simulink model "q_find_deadzone"  (R2014a)
settings: Solver=ode1  StartTime=0.0  StopTime=inf  FixedStep=0.001  RelTol=1e-3
undefined symbols (not defined in the file or in its folder): HIL
libraries: quarc_library x4
settings Model: SimulationMode=external  ExtModeTrigDuration=30000  Creator=Student  LastModifiedBy=Control_Eng
settings SolverCC: PositivePriorityOrder=on
settings RTWCC: SystemTargetFile=quarc_win64.tlc  TemplateMakefile=quarc_default_tmf  Description=QUARC Win64 Target  ProcessScript=quarc_win64_make_rtw_hook
settings STFCustomTargetCC: CombineOutputUpdateFcns=on  GRTInterface=off
settings GRTTargetCC: ParMdlRefBuildCompliant=off  CompOptLevelCompliant=off  MatFileLogging=off  CPPClassGenCompliant=off  ExtMode=on  ExtModeMexFile=quarc_comm

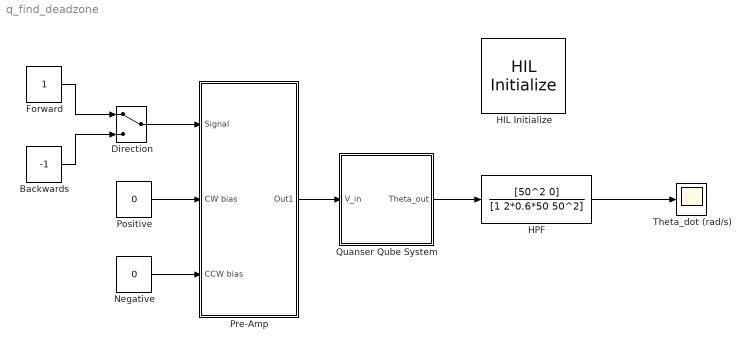
== system q_find_deadzone ==
  Backwards : Constant  Value=-1
  Direction : ManualSwitch
  Forward : Constant
  HIL Initialize : quarc_library/Data Acquisition/Generic/Configuration/HIL Initialize  Priority=-99  object_name=HIL-1  board_type=qube_servo_usb  board_number=0  board_options=d0=pwm;d1=pwm;led=auto;update_rate=normal;decimation=1  exclusive=off  active=off  hardware_clocks=[0]  clock_modes=[]  initial_clock_frequencies=[]  set_clock_params_at_start=off  set_clock_params_at_switch_in=off  set_clock_frequencies_at_start=off  set_clock_frequencies_at_switch_in=off  analog_input_channels=[]  analog_input_maximums=[]  analog_input_minimums=[]  set_analog_input_params_at_start=off  set_analog_input_params_at_switch_in=off  analog_output_channels=[0:1]  analog_output_maximums=10  analog_output_minimums=-10  initial_analog_outputs=[0]  final_analog_outputs=[0]  watchdog_analog_outputs=0  set_analog_output_params_at_start=on  set_analog_output_params_at_switch_in=off  set_analog_outputs_at_start=on  set_analog_outputs_at_switch_in=off  set_analog_outputs_at_terminate=on  set_analog_outputs_at_switch_out=off  set_analog_outputs_on_watchdog=off  digital_input_channels=[]  digital_output_channels=[]  digital_output_configuration=[]  initial_digital_outputs=[]  final_digital_outputs=[]  watchdog_digital_outputs=[]  set_digital_output_params_at_start=off  set_digital_output_params_at_switch_in=off  set_digital_outputs_at_start=off  set_digital_outputs_at_switch_in=off  set_digital_outputs_at_terminate=off  set_digital_outputs_at_switch_out=off  set_digital_outputs_on_watchdog=off  encoder_channels=[0:1]  quadrature=[4]  encoder_filter_frequency=[]  initial_encoder_counts=[0]  set_encoder_params_at_start=on  set_encoder_params_at_switch_in=off  set_encoder_counts_at_start=on  set_encoder_counts_at_switch_in=off  pwm_channels=[]  pwm_modes=[]  pwm_frequency=[]  pwm_configuration=[]  pwm_alignment=[]  pwm_polarity=[]  pwm_leading_deadband=[]  pwm_trailing_deadband=[]  initial_pwm_outputs=[]  final_pwm_outputs=[]  watchdog_pwm_outputs=[]  set_pwm_params_at_start=off  set_pwm_params_at_switch_in=off  set_pwm_outputs_at_start=off  set_pwm_outputs_at_switch_in=off  set_pwm_outputs_at_terminate=off  set_pwm_outputs_at_switch_out=off  set_pwm_outputs_on_watchdog=off  other_output_channels=[]  initial_other_outputs=[]  final_other_outputs=[]  watchdog_other_outputs=[]  set_other_outputs_at_start=off  set_other_outputs_at_switch_in=off  set_other_outputs_at_terminate=off  set_other_outputs_at_switch_out=off  set_other_outputs_on_watchdog=off
  HPF : TransferFcn  Numerator=[50^2 0]  Denominator=[1 2*0.6*50 50^2]
  Negative : Constant  Value=0
  Positive : Constant  Value=0
  Pre-Amp : Subsystem
  Quanser Qube System : Subsystem
  Theta_dot (rad/s) : Scope
      settings: TimeRange=30  YMin=0  YMax=50  SaveName=Output_Data  MaxDataPoints=2500
  wires:
  Quanser Qube System/1(Theta_out) -> HPF/1
  Positive/1 -> Pre-Amp/2(CW bias)
  Negative/1 -> Pre-Amp/3(CCW bias)
  Pre-Amp/1(Out1) -> Quanser Qube System/1(V_in)
  HPF/1 -> Theta_dot (rad/s)/1
  Direction/1 -> Pre-Amp/1(Signal)
  Backwards/1 -> Direction/2
  Forward/1 -> Direction/1

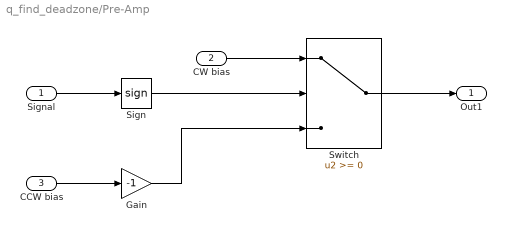
== system q_find_deadzone/Pre-Amp ==
  Signal : Inport
  CW bias : Inport  Port=2
  CCW bias : Inport  Port=3
  Gain : Gain  Gain=-1
  Sign : Signum
  Switch : Switch
  Out1 : Outport
  wires:
  CW bias/1 -> Switch/1
  Signal/1 -> Sign/1
  CCW bias/1 -> Gain/1
  Switch/1 -> Out1/1
  Sign/1 -> Switch/2
  Gain/1 -> Switch/3

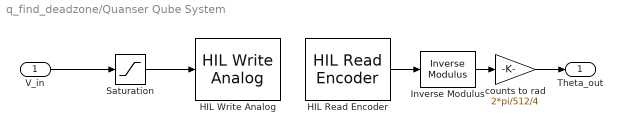
== system q_find_deadzone/Quanser Qube System ==
  V_in : Inport
  HIL Read Encoder : quarc_library/Data Acquisition/Generic/Immediate I//O/HIL Read Encoder  object_name=HIL-1  channels=0  sample_time=qc_get_step_size  active=on  vector_output=off  data_type_mode=Inherit via back propagation  data_type=double
  HIL Write Analog : quarc_library/Data Acquisition/Generic/Immediate I//O/HIL Write Analog  object_name=HIL-1  channels=0  sample_time=-1  active=off  vector_input=off
  Inverse Modulus : quarc_library/Discontinuities/Inverse Modulus  modulus=2^16  output_derivative=off  output_revolutions=off  max_x=Inf  min_x=-Inf
  Saturation : Saturate  UpperLimit=6  LowerLimit=-6
  counts to rad : Gain  Gain=2*pi/512/4
  Theta_out : Outport
  wires:
  V_in/1 -> Saturation/1
  HIL Read Encoder/1 -> Inverse Modulus/1
  Inverse Modulus/1 -> counts to rad/1
  counts to rad/1 -> Theta_out/1
  Saturation/1 -> HIL Write Analog/1
